simulink library "tqd"  (R2021b)
settings: Solver=VariableStepAuto  StartTime=0.0  StopTime=10.0  RelTol=1e-3
undefined symbols (not defined in the file): ATQD_AfterTqMinGain_X_Deg, ATQD_APSCreepBaseTqD_X_kph, ATQD_APSCreepBaseTqD_Y_Deg, ATQD_APSCreepBaseTqR_X_kph, ATQD_APSCreepBaseTqR_Y_Deg, ATQD_APSCreepIterm_X_kph, ATQD_APSCreepIterm_Y_kph, ATQD_APSCreepPterm_X_kph, ATQD_APSCreepPterm_Y_kph, ATQD_APSDecReq_X_kph, ATQD_APSDecReq_Y_mps2, ATQD_APSDecReqCMD_X_kph, ATQD_APSDecReqTs_X_pct, ATQD_APSDecTimeGain_X_Deg, ATQD_APSDecTimeGain_Y_s, ATQD_APSReqLowSpd_X_Deg, ATQD_AutoHoldReleaseBPS_X_Deg, ATQD_AWDLoadTrqnsGain_X_kg, ATQD_AWDLoadTrqnsGain_Y_pct, ATQD_BOSEnBPSPosn_X_kph, ATQD_BOSMap_X_rpm, ATQD_BOSMap_Y_pct, ATQD_CreepBaseTqD_X_kph, ATQD_CreepBaseTqD_Y_Deg, ATQD_CreepBaseTqR_X_kph, ATQD_CreepBaseTqR_Y_Deg, ATQD_CreepBPSDisPosn_X_Deg, ATQD_CreepBPSDisPosnR_X_Deg, ATQD_CreepBPSEnPosn_X_Deg, ATQD_CreepBPSEnPosnR_X_Deg, ATQD_CreepDeltaTq_X_kph, ATQD_CreepIterm_X_kph, ATQD_CreepIterm_Y_kph, ATQD_CreepItermMaxLimit_X_pct, ATQD_CreepPreloadTime_X_kph, ATQD_CreepPreloadTq_X_kph, ATQD_CreepPreloadTq_Y_s, ATQD_CreepProtTq_X_Deg, ATQD_CreepPterm_X_kph, ATQD_CreepPterm_Y_kph, ATQD_CreepRrTqSpRat_X_rpm, ATQD_CreepRrTqSpRat_Y_Nm, ATQD_CreepTargetSpdD_X_pct, ATQD_CreepTargetSpdR_X_pct, ATQD_ECOTqMapD_X_rpm, ATQD_ECOTqMapD_Y_pct, ATQD_EMTqMapD_X_rpm, ATQD_EMTqMapD_Y_pct, ATQD_EOPDTqMapDCon_X_rpm, ATQD_EOPDTqMapDCon_Y_Deg, ATQD_EscapeModePedTq_X_pct, ATQD_EscapeModePedTq_Y_rpm, ATQD_EscapeModePedTqFr_X_pct, ATQD_EscapeModePedTqFr_Y_rpm, ATQD_EstInitVehWeight_X_c, ATQD_FAfterTqCMDGain_X_rpm, ATQD_FAfterTqCMDGain_Y_pct, ATQD_FrLossMAPLowV_X_rpm, ATQD_FrLossMAPLowV_Y_Nm, ATQD_FrMotActReduce_X_rpm ... (+772)
libraries: simulink x211, hcu_lib x179, tqr x3
(part 13 of 28)

== system tqd/TQD/TorqueDemand/Signal_convert/VehWeightEst/Condition ==
  VTQD_AfterAvailableTqDemRr_Nm : Inport
  VTQR_NoABSREDUWhlTqReq_Nm : Inport  Port=2
  VTQR_NoABSFEDUWhlTqReq_Nm : Inport  Port=3
  VTQD_AfterAvailableTqDemFr_Nm : Inport  Port=4
  VTQD_GearActualPosn_enum : Inport  Port=5
  VINP_VehSpeed_kph : Inport  Port=6
  VTQD_RollRegenDisableReq_flg : Inport  Port=7
  VINP_RegenMode_enum : Inport  Port=8
  VTQD_LowIdleAccPedal_flg : Inport  Port=9
  VTQD_BrkSwSta_flg : Inport  Port=10
  VINP_RrRBCActive_flg : Inport  Port=11
  VINP_FrRBCActive_flg : Inport  Port=12
  VINP_GRADE_Deg : Inport  Port=13
  task_time_s : Inport  Port=14
  VTQD_VehWeightEstEnd_flg : Inport  Port=15
  AND1 : Logic  Inputs=13  AllPortsSameDT=off  OutDataTypeStr=boolean
  Abs : Abs
  Abs1 : Abs
  Abs2 : Abs
  Add : Sum  Inputs=+-
  Add1 : Sum  Inputs=+-
  Constant1 : Constant  Value=KTQD_VehWeightEstSpdEnLow_kph
  Constant10 : Constant  Value=eps
  Constant11 : Constant  Value=KTQD_VehWeightEstSpdEnUp_kph
  Constant2 : Constant  Value=ENUM_REGENLEVEL_LV1
  Constant3 : Constant  Value=KTQD_RrTqDeviation_Nm
  Constant4 : Constant  Value=KTQD_FrTqDeviation_Nm
  Constant5 : Constant  Value=KTQD_VehWeightEstGradeEn_Deg
  Constant6 : Constant  Value=KTQD_VehWeighEstTime_s
  Constant7 : Constant  Value=KTQD_EstDelayEnTime_s
  Constant8 : Constant  Value=KTQD_EstWeighResetTime_s
  Constant9 : Constant  Value=ENUM_GEARACTUALPOSN_D
  Delay{,1..5} (6 alike) : Delay  DelayLength=1
  DelayEnable : hcu_lib/Basic_Blocks/DelayEnable
  Detect Increase : simulink/Logic and Bit Operations/Detect Increase  vinit=0.0  OutDataTypeStr=boolean
  Equal : RelationalOperator  Operator=<  OutDataTypeStr=boolean  RndMeth=Simplest
  Equal1 : RelationalOperator  Operator===  OutDataTypeStr=boolean  RndMeth=Simplest
  Equal2 : RelationalOperator  Operator=~=  OutDataTypeStr=boolean  RndMeth=Simplest
  Less Than1 : RelationalOperator  Operator=<  OutDataTypeStr=boolean  RndMeth=Simplest
  Less Than2 : RelationalOperator  Operator=>  OutDataTypeStr=boolean  RndMeth=Simplest
  Less Than3 : RelationalOperator  Operator=<=  OutDataTypeStr=boolean  RndMeth=Simplest
  Less Than4 : RelationalOperator  Operator=<=  OutDataTypeStr=boolean  RndMeth=Simplest
  Less Than5 : RelationalOperator  Operator=<=  OutDataTypeStr=boolean  RndMeth=Simplest
  NOT{,1..5} (6 alike) : Logic  Operator=NOT  AllPortsSameDT=off  OutDataTypeStr=boolean
  Relational Operator : RelationalOperator  OutDataTypeStr=boolean  RndMeth=Simplest
  Relational Operator1 : RelationalOperator  OutDataTypeStr=boolean  RndMeth=Simplest
  SR_Latch : hcu_lib/Basic_Blocks/SR_Latch
  Timer : hcu_lib/Basic_Blocks/Timer
  Timer1 : hcu_lib/Basic_Blocks/Timer
  VTQD_VehWeightEstEn_flg : Outport
  VTQD_VehWeightEstDis_flg : Outport  Port=2
  wires:
  Constant9/1 -> Equal1/2
  Less Than1/1 -> AND1/2  "VTQD_VehWeightEstEnCon2_flg"
  Abs/1 -> [VTQD_RrTqErr_Nm]  "VTQD_RrTqErr_Nm"
  Equal1/1 -> AND1/1  "VTQD_VehWeightEstEnCon1_flg"
  Constant11/1 -> Less Than1/2
  [VTQR_NoABSFEDUWhlTqReq_Nm] -> Delay1/1
  Constant4/1 -> Less Than4/2
  Add1/1 -> Abs1/1
  [VTQD_RollRegenDisableReq_flg] -> NOT/1
  [VTQD_RrTqErr_Nm] -> Less Than3/1
  Add/1 -> Abs/1
  [VTQD_BrkSwSta_flg] -> NOT3/1
  [VTQD_FrTqErr_Nm] -> Less Than4/1
  Abs1/1 -> [VTQD_FrTqErr_Nm]  "VTQD_FrTqErr_Nm"
  [VTQD_GearActualPosn_enum] -> Equal1/1
  [VINP_VehSpeed_kph] -> Less Than1/1
  [VINP_RegenMode_enum] -> Equal2/1
  [VTQD_AfterAvailableTqDemFr_Nm] -> Delay4/1
  Constant1/1 -> Less Than2/2
  [VTQD_AfterAvailableTqDemRr_Nm] -> Delay2/1
  Less Than4/1 -> AND1/8  "VTQD_VehWeightEstEnCon7_flg"
  [VINP_RrRBCActive_flg] -> NOT4/1
  [VTQR_NoABSREDUWhlTqReq_Nm] -> Delay3/1
  NOT/1 -> AND1/4  "VTQD_VehWeightEstEnCon4_flg"
  [VINP_FrRBCActive_flg] -> NOT5/1
  Constant5/1 -> Less Than5/2
  Equal2/1 -> AND1/5  "VTQD_VehWeightEstEnCon5_flg"
  [VTQD_LowIdleAccPedal_flg] -> AND1/6
  Constant2/1 -> Equal2/2
  Less Than3/1 -> AND1/7  "VTQD_VehWeightEstEnCon6_flg"
  Less Than2/1 -> AND1/3  "VTQD_VehWeightEstEnCon3_flg"
  [VINP_VehSpeed_kph] -> Less Than2/1
  Less Than5/1 -> AND1/12  "VTQD_VehWeightEstEnCon11_flg"
  [VINP_GRADE_Deg] -> Abs2/1
  Abs2/1 -> Less Than5/1
  Constant3/1 -> Less Than3/2
  VTQD_AfterAvailableTqDemRr_Nm/1 -> [VTQD_AfterAvailableTqDemRr_Nm]
  VTQR_NoABSREDUWhlTqReq_Nm/1 -> [VTQR_NoABSREDUWhlTqReq_Nm]
  VTQD_AfterAvailableTqDemFr_Nm/1 -> [VTQD_AfterAvailableTqDemFr_Nm]
  VTQR_NoABSFEDUWhlTqReq_Nm/1 -> [VTQR_NoABSFEDUWhlTqReq_Nm]
  VTQD_GearActualPosn_enum/1 -> [VTQD_GearActualPosn_enum]
  VINP_VehSpeed_kph/1 -> [VINP_VehSpeed_kph]
  VTQD_RollRegenDisableReq_flg/1 -> [VTQD_RollRegenDisableReq_flg]
  VINP_RegenMode_enum/1 -> [VINP_RegenMode_enum]
  VTQD_LowIdleAccPedal_flg/1 -> [VTQD_LowIdleAccPedal_flg]
  VTQD_BrkSwSta_flg/1 -> [VTQD_BrkSwSta_flg]
  VINP_RrRBCActive_flg/1 -> [VINP_RrRBCActive_flg]
  VINP_FrRBCActive_flg/1 -> [VINP_FrRBCActive_flg]
  VINP_GRADE_Deg/1 -> [VINP_GRADE_Deg]
  [VTQD_VehWeightEstEn_flg] -> VTQD_VehWeightEstEn_flg/1
  Relational Operator/1 -> [VTQD_VehWeightEstDis_flg]  "VTQD_VehWeightEstDis_flg"
  Timer/1 -> Relational Operator/1
  NOT1/1 -> Timer/2
  [VTQD_VehWeightEstEn_flg] -> NOT1/1, Timer/1
  Constant6/1 -> Relational Operator/2, Timer/4
  [VTQD_VehWeightEstDis_flg] -> VTQD_VehWeightEstDis_flg/1
  task_time_s/1 -> [task_time_s]
  AND1/1 -> DelayEnable/1
  DelayEnable/1 -> [VTQD_VehWeightEstEn_flg]  "VTQD_VehWeightEstEn_flg"
  [task_time_s] -> DelayEnable/3
  Constant7/1 -> DelayEnable/2
  [VTQD_VehWeightEstEnd_flg] -> Detect Increase/1
  Detect Increase/1 -> SR_Latch/1
  SR_Latch/1 -> NOT2/1, Timer1/1
  NOT2/1 -> Timer1/2
  Constant8/1 -> Relational Operator1/2, Timer1/4
  Timer1/1 -> [VTQD_EstVehWeightResetTime_s], Relational Operator1/1  "VTQD_EstVehWeightResetTime_s"
  Relational Operator1/1 -> [VTQD_EstVehWeitResetFinish_flg]  "VTQD_EstVehWeitResetFinish_flg"
  [VTQD_EstVehWeitResetFinish_flg] -> Delay/1
  Delay/1 -> SR_Latch/2
  [VTQD_EstVehWeightResetTime_s] -> Delay5/1
  Constant10/1 -> Equal/2
  Equal/1 -> AND1/13  "VTQD_VehWeightEstEnCon12_flg"
  VTQD_VehWeightEstEnd_flg/1 -> [VTQD_VehWeightEstEnd_flg]
  Delay1/1 -> Add1/1
  Delay2/1 -> Add/1
  Delay3/1 -> Add/2
  Delay4/1 -> Add1/2
  Delay5/1 -> Equal/1
  NOT3/1 -> AND1/9  "VTQD_VehWeightEstEnCon8_flg"
  NOT4/1 -> AND1/10  "VTQD_VehWeightEstEnCon9_flg"
  NOT5/1 -> AND1/11  "VTQD_VehWeightEstEnCon10_flg"
  [task_time_s] -> Timer/3
  [task_time_s] -> Timer1/3

== system tqd/TQD/TorqueDemand/Signal_convert/VehWeightEst/Desicion ==
  task_time_s : Inport
  VTQD_VehWeightEstDis_flg : Inport  Port=2
  VTQD_EstVehWeight_kg : Inport  Port=3
  VINP_DriverSeatBeltCmd_flg : Inport  Port=4
  VINP_PsngrSeatBeltCmd_flg : Inport  Port=5
  VINP_RDriverSeatBeltCmd_flg : Inport  Port=6
  VINP_RCenterSeatBeltCmd_flg : Inport  Port=7
  VINP_RPsngrSeatBeltCmd_flg : Inport  Port=8
  VTQD_EstLongAccCheckPass_flg : Inport  Port=9
  VTQD_EstFrRealTqCheckPass_flg : Inport  Port=10
  VTQD_EstRrRealTqCheckPass_flg : Inport  Port=11
  AND : Logic  Inputs=5  AllPortsSameDT=off  OutDataTypeStr=boolean
  Add : Sum  Inputs=+++++
  Constant1 : Constant  Value=eps
  Constant{2,4,6,8,10} (5 alike) : Constant  Value=ZERO_INT
  Constant{3,5,7,9,11} (5 alike) : Constant  Value=ONE_INT
  Constant12 : Constant  Value=KTQD_EstEndDelayTime_s
  Data Type Conversion : DataTypeConversion  OutDataTypeStr=single
  Delay : Delay  DelayLength=1
  Delay1 : Delay  DelayLength=1
  DelayEnable : hcu_lib/Basic_Blocks/DelayEnable
  Equal : RelationalOperator  OutDataTypeStr=boolean  RndMeth=Simplest
  MTQD_EstInitVehWeight_Y_kg : Lookup_n-D  NumberOfTableDimensions=1  BreakpointsForDimension1=ATQD_EstInitVehWeight_X_c  Table=MTQD_EstInitVehWeight_Y_kg  ExtrapMethod=Clip  InternalRulePriority=Speed  RndMeth=Simplest  InputSameDT=on
  NOT : Logic  Operator=NOT  AllPortsSameDT=off  OutDataTypeStr=boolean
  Switch{,1..6} (7 alike) : Switch  Criteria=u2 > Threshold
  VTQD_VehWeightEstEnd_flg : Outport
  VTQD_EstVehWeightResult_kg : Outport  Port=2
  wires:
  Constant7/1 -> Switch4/1
  Constant1/1 -> Equal/2
  Switch2/1 -> Add/1
  [VINP_DriverSeatBeltCmd_flg] -> Switch2/2
  [VINP_RCenterSeatBeltCmd_flg] -> Switch4/2
  Switch5/1 -> Add/4
  Equal/1 -> Switch1/2
  Constant10/1 -> Switch6/3
  [VTQD_VehWeightEstDis_flg] -> AND/1
  Switch6/1 -> Add/5
  Delay/1 -> NOT/1
  Switch3/1 -> Add/2
  Constant6/1 -> Switch4/3
  Constant3/1 -> Switch2/1
  [VTQD_EstActVehWeight_kg] -> Switch1/1
  Constant2/1 -> Switch2/3
  [VTQD_VehWeightEstEnter_flg] -> Switch/2
  Constant11/1 -> Switch6/1
  Switch1/1 -> [VTQD_EstVehWeightResult_kg]  "VTQD_EstVehWeightResult_kg"
  Constant4/1 -> Switch3/3
  Constant5/1 -> Switch3/1
  [VINP_RDriverSeatBeltCmd_flg] -> Switch5/2
  Switch/1 -> Delay1/1, [VTQD_EstActVehWeight_kg]  "VTQD_EstActVehWeight_kg"
  AND/1 -> [VTQD_VehWeightEstEnter_flg]  "VTQD_VehWeightEstEnter_flg"
  [VINP_RPsngrSeatBeltCmd_flg] -> Switch6/2
  [VTQD_EstActVehWeight_kg] -> Equal/1
  [VINP_PsngrSeatBeltCmd_flg] -> Switch3/2
  Delay1/1 -> Switch/3
  [VTQD_EstInitVehWeight_kg] -> Switch1/3
  Constant9/1 -> Switch5/1
  Constant8/1 -> Switch5/3
  [VTQD_EstVehWeight_kg] -> Switch/1
  [VTQD_VehWeightEstEnd_flg] -> Delay/1
  NOT/1 -> AND/2
  Switch4/1 -> Add/3
  [VTQD_VehWeightEstDis_flg] -> DelayEnable/1
  Constant12/1 -> DelayEnable/2
  [task_time_s] -> DelayEnable/3
  DelayEnable/1 -> [VTQD_VehWeightEstEnd_flg]  "VTQD_VehWeightEstEnd_flg"
  task_time_s/1 -> [task_time_s]
  [VTQD_VehWeightEstEnd_flg] -> VTQD_VehWeightEstEnd_flg/1
  VTQD_VehWeightEstDis_flg/1 -> [VTQD_VehWeightEstDis_flg]
  VTQD_EstVehWeight_kg/1 -> [VTQD_EstVehWeight_kg]
  [VTQD_EstVehWeightResult_kg] -> VTQD_EstVehWeightResult_kg/1
  VINP_DriverSeatBeltCmd_flg/1 -> [VINP_DriverSeatBeltCmd_flg]
  VINP_PsngrSeatBeltCmd_flg/1 -> [VINP_PsngrSeatBeltCmd_flg]
  VINP_RDriverSeatBeltCmd_flg/1 -> [VINP_RDriverSeatBeltCmd_flg]
  VINP_RCenterSeatBeltCmd_flg/1 -> [VINP_RCenterSeatBeltCmd_flg]
  VINP_RPsngrSeatBeltCmd_flg/1 -> [VINP_RPsngrSeatBeltCmd_flg]
  VTQD_EstRrRealTqCheckPass_flg/1 -> [VTQD_EstRrRealTqCheckPass_flg]
  VTQD_EstFrRealTqCheckPass_flg/1 -> [VTQD_EstFrRealTqCheckPass_flg]
  VTQD_EstLongAccCheckPass_flg/1 -> [VTQD_EstLongAccCheckPass_flg]
  [VTQD_EstLongAccCheckPass_flg] -> AND/3
  [VTQD_EstFrRealTqCheckPass_flg] -> AND/4
  [VTQD_EstRrRealTqCheckPass_flg] -> AND/5
  MTQD_EstInitVehWeight_Y_kg/1 -> [VTQD_EstInitVehWeight_kg]  "VTQD_EstInitVehWeight_kg"
  Data Type Conversion/1 -> MTQD_EstInitVehWeight_Y_kg/1
  Add/1 -> Data Type Conversion/1  "VTQD_EstInitVehWightX_c"

== system tqd/TQD/TorqueDemand/TorqueModule/AvaliableTqLimit/If Action Subsystem1 ==
  VTQD_WhlTqCapGenF_Nm : Inport
  VTQD_WhlTqCapGenR_Nm : Inport  Port=2
  VTQD_DriverWhlTqDemFr_Nm : Inport  Port=3
  VTQD_DriverWhlTqDemRr_Nm : Inport  Port=4
  VVMC_ADASActive_flg : Inport  Port=5
  Action Port : ActionPort
  Constant{,1..3} (4 alike) : Constant  Value=ZERO_FLOAT
  Data Type Conversion1 : DataTypeConversion  OutDataTypeStr=single
  Data Type Conversion5 : DataTypeConversion  OutDataTypeStr=single
  Display : Display
  Display1 : Display
  Subtract : Sum  Inputs=+-
  Subtract1 : Sum  Inputs=+-
  Switch : Switch  Criteria=u2 > Threshold
  Switch1 : Switch  Criteria=u2 > Threshold
  Switch2 : Switch  Criteria=u2 ~= 0
  Switch3 : Switch  Criteria=u2 ~= 0
  VTQD_AvailTqWithARgnFr_Nm : Outport
  VTQD_AvailTqWithARgnRr_Nm : Outport  Port=2
  wires:
  Constant1/1 -> Switch1/1
  Constant/1 -> Switch/1
  Subtract1/1 -> Switch1/2, Switch1/3
  Subtract/1 -> Switch/2, Switch/3
  Switch1/1 -> Data Type Conversion5/1, VTQD_AvailTqWithARgnRr_Nm/1
  Switch/1 -> Data Type Conversion1/1, VTQD_AvailTqWithARgnFr_Nm/1
  VTQD_WhlTqCapGenR_Nm/1 -> Subtract1/1
  VTQD_WhlTqCapGenF_Nm/1 -> Subtract/1
  VTQD_DriverWhlTqDemFr_Nm/1 -> Switch2/3
  Switch2/1 -> Subtract/2
  Constant2/1 -> Switch2/1
  VVMC_ADASActive_flg/1 -> Switch3/2, Switch2/2
  Constant3/1 -> Switch3/1
  VTQD_DriverWhlTqDemRr_Nm/1 -> Switch3/3
  Switch3/1 -> Subtract1/2
  Data Type Conversion1/1 -> Display/1  "VTQD_AvailTqWithARgnFr_Nm"
  Data Type Conversion5/1 -> Display1/1  "VTQD_AvailTqWithARgnRr_Nm"

== system tqd/TQD/TorqueDemand/TorqueModule/AvaliableTqLimit/If Action Subsystem2 ==
  VTQD_WhlTqCapGenF_Nm : Inport
  VTQD_WhlTqCapGenR_Nm : Inport  Port=2
  Action Port : ActionPort
  Data Type Conversion4 : DataTypeConversion  OutDataTypeStr=single
  Data Type Conversion5 : DataTypeConversion  OutDataTypeStr=single
  Display : Display
  Display1 : Display
  VTQD_AvailTqNoARgnFr_Nm : Outport
  VTQD_AvailTqNoARgnRr_Nm : Outport  Port=2
  wires:
  VTQD_WhlTqCapGenF_Nm/1 -> Data Type Conversion4/1, VTQD_AvailTqNoARgnFr_Nm/1
  VTQD_WhlTqCapGenR_Nm/1 -> Data Type Conversion5/1, VTQD_AvailTqNoARgnRr_Nm/1
  Data Type Conversion4/1 -> Display/1  "VTQD_AvailTqNoARgnFr_Nm"
  Data Type Conversion5/1 -> Display1/1  "VTQD_AvailTqNoARgnRr_Nm"

== system tqd/TQD/TorqueDemand/TorqueModule/AvaliableTqLimit/TorqueCapacityCalcalation ==
  VTQD_FrShaftSpd_rpm : Inport
  VTQD_RrShaftSpd_rpm : Inport  Port=2
  VINP_HVBPwrAvailDchrg_kw : Inport  Port=3
  VINP_HVBPwrAvailChrg_kw : Inport  Port=4
  KTQD_FrBatapCont_factor : Inport  Port=5
  KTQD_RrBatapCont_factor : Inport  Port=6
  VTQD_FrEDUSpRat_cmd : Inport  Port=7
  VTQD_RrEDUSpRat_rat : Inport  Port=8
  VINP_FrMotorAvailTq_Nm : Inport  Port=9
  VINP_RrMotorAvailTq_Nm : Inport  Port=10
  VINP_FrRegenAvailTq_Nm : Inport  Port=11
  VINP_RrRegenAvailTq_Nm : Inport  Port=12
  VTQD_GearActualPosn_enum : Inport  Port=13
  VINP_VehicleType_enum : Inport  Port=14
  VTQD_CoordWhlTqDemFr_Nm : Inport  Port=15
  VTQD_CoordWhlTqDemRr_Nm : Inport  Port=16
  VINP_FrMCUDCBusVolt_V : Inport  Port=17
  VINP_RrMCUDCBusVolt_V : Inport  Port=18
  VPMM_DrivetrainSelect_enum : Inport  Port=19
  VINP_FrMCUTemp_C : Inport  Port=20
  VINP_FrTMTemp_C : Inport  Port=21
  VINP_RrMCUTemp_C : Inport  Port=22
  VINP_RrTMTemp_C : Inport  Port=23
  VTQD_IVIRockModeEn_flg : Inport  Port=24
  VTQD_ActAPSPosn_pct : Inport  Port=25
  task_time_s : Inport  Port=26
  CapacityDistribution : Subsystem
  Constant1 : Constant  Value=KTQD_RockInitMotTqInc_Nm
  Constant10 : Constant  Value=KTQD_RrUppTheldTrq_Nm
  Constant11 : Constant  Value=KTQD_RrUppTheldTrq_Nm
  Constant12 : Constant  Value=KTQD_RockInitTqMotDec_Nm
  Constant13 : Constant  Value=KTQD_RockAvalMotTqReset_pct
  Constant14 : Constant  Value=KTQD_RockAvalMotTqReset_pct
  Constant2 : Constant  Value=KTQD_FrRockAvalMotTqInc_Nm
  Constant3 : Constant  Value=KTQD_FrRockAvalMotBaseTq_Nm
  Constant4 : Constant  Value=KTQD_FrUppTheldTrq_Nm
  Constant5 : Constant  Value=KTQD_FrUppTheldTrq_Nm
  Constant6 : Constant  Value=KTQD_RockInitTqMotDec_Nm
  Constant7 : Constant  Value=KTQD_RockInitMotTqInc_Nm
  Constant8 : Constant  Value=KTQD_RrRockAvalMotTqInc_Nm
  Constant9 : Constant  Value=KTQD_RrRockAvalMotBaseTq_Nm
  Generation : Subsystem
  KTQD_FrMotorTempHigh_C KTQD_FrMotorTempLow_C : Relay  OnSwitchValue=KTQD_FrMotorTempHigh_C  OffSwitchValue=KTQD_FrMotorTempLow_C  OutDataTypeStr=boolean
  KTQD_RrMotorTempHigh_C KTQD_RrMotorTempLow_C : Relay  OnSwitchValue=KTQD_RrMotorTempHigh_C  OffSwitchValue=KTQD_RrMotorTempLow_C  OutDataTypeStr=boolean
  "MOTOR Loss MAP " : Subsystem
  MTQD_FrGenActReduce_Z_Nm : Lookup_n-D  BreakpointsForDimension1=ATQD_FrMotActReduce_Y_C  BreakpointsForDimension2=ATQD_FrMotActReduce_X_rpm  Table=MTQD_FrGenActReduce_Z_Nm  InternalRulePriority=Speed  RndMeth=Simplest  InputSameDT=on
      settings: InputPortMap=u0,u1
  MTQD_FrMotActReduce_Z_Nm : Lookup_n-D  BreakpointsForDimension1=ATQD_FrMotActReduce_Y_C  BreakpointsForDimension2=ATQD_FrMotActReduce_X_rpm  Table=MTQD_FrMotActReduce_Z_Nm  InternalRulePriority=Speed  RndMeth=Simplest  InputSameDT=on
      settings: InputPortMap=u0,u1
  MTQD_RrGenActReduce_Z_Nm : Lookup_n-D  BreakpointsForDimension1=ATQD_FrMotActReduce_Y_C  BreakpointsForDimension2=ATQD_FrMotActReduce_X_rpm  Table=MTQD_RrGenActReduce_Z_Nm  InternalRulePriority=Speed  RndMeth=Simplest  InputSameDT=on
      settings: InputPortMap=u0,u1
  MTQD_RrMotActReduce_Z_Nm : Lookup_n-D  BreakpointsForDimension1=ATQD_FrMotActReduce_Y_C  BreakpointsForDimension2=ATQD_FrMotActReduce_X_rpm  Table=MTQD_RrMotActReduce_Z_Nm  InternalRulePriority=Speed  RndMeth=Simplest  InputSameDT=on
      settings: InputPortMap=u0,u1
  Max{,1..7} (8 alike) : MinMax  Function=max  Inputs=2
  Motoring : Subsystem
  OR : Logic  Operator=OR  AllPortsSameDT=off  OutDataTypeStr=boolean
  OR1 : Logic  Operator=OR  AllPortsSameDT=off  OutDataTypeStr=boolean
  RateLimit : hcu_lib/Basic_Blocks/RateLimit
  RateLimit1 : hcu_lib/Basic_Blocks/RateLimit
  Relational Operator : RelationalOperator  Operator=<=  OutDataTypeStr=boolean  RndMeth=Simplest
  Relational Operator1 : RelationalOperator  Operator=<=  OutDataTypeStr=boolean  RndMeth=Simplest
  Switch{,1..3} (4 alike) : Switch  Criteria=u2 ~= 0
      settings: AttributesFormatString=%<Criteria>
  TMAvailablePwr_Calculation : Subsystem
  VTQD_WhlTqCapMotFr_Nm : Outport
  VTQD_WhlTqCapMotRr_Nm : Outport  Port=2
  VTQD_WhlTqCapGenFr_Nm : Outport  Port=3
  VTQD_WhlTqCapGenRr_Nm : Outport  Port=4
  VTQD_MotorLossTotal_kw : Outport  Port=5
  wires:
  [VTQD_TMPwrAvailDchrg_kW] -> CapacityDistribution/3(VTQD_TMPwrAvailDchrg_kW)
  TMAvailablePwr_Calculation/1(VTQD_TMPwrAvailDchrg_kW) -> [VTQD_TMPwrAvailDchrg_kW]
  [VINP_HVBPwrAvailDchrg_kw] -> TMAvailablePwr_Calculation/1(VINP_HVBPwrAvailDchrg_kw)
  Motoring/2(VTQD_WhlTqCapMotRr_Nm) -> VTQD_WhlTqCapMotRr_Nm/1
  [VTQD_RrEDUSpRat_rat] -> CapacityDistribution/2(VTQD_RrEDUSpRat_rat)
  [VTQD_FrEDUSpRat_rat] -> CapacityDistribution/1(VTQD_FrEDUSpRat_cmd)
  CapacityDistribution/4(VTQD_RrHVBPwrAvailChrg_kw) -> [VTQD_RrHVBPwrAvailChrg_kw]
  CapacityDistribution/3(VTQD_FrHVBPwrAvailChrg_kw) -> [VTQD_FrHVBPwrAvailChrg_kw]
  CapacityDistribution/2(VTQD_RrHVBPwrAvailDchrg_kw) -> [VTQD_RrHVBPwrAvailDchrg_kw]
  CapacityDistribution/1(VTQD_FrHVBPwrAvailDchrg_kw) -> [VTQD_FrHVBPwrAvailDchrg_kw]
  [VINP_HVBPwrAvailChrg_kw] -> CapacityDistribution/4(VINP_HVBPwrAvailChrg_kw)
  [VTQD_RrHVBPwrAvailChrg_kw] -> Generation/4(VTQD_RrHVBPwrAvailChrg_kw)
  [KTQD_RrBatapCont_factor] -> Generation/6(KTQD_RrBatapCont_factor)
  [VTQD_FrShaftSpd_rpm] -> Generation/1(VTQD_FrShaftSpd_rpm)
  [VTQD_FrHVBPwrAvailChrg_kw] -> Generation/3(VTQD_FrHVBPwrAvailChrg_kw)
  [VTQD_RrShaftSpd_rpm] -> Generation/2(VTQD_RrShaftSpd_rpm)
  [KTQD_FrBatapCont_factor] -> Generation/5(KTQD_FrBatapCont_factor)
  Generation/1(VTQD_WhlTqCapGenFr_Nm) -> VTQD_WhlTqCapGenFr_Nm/1
  Generation/2(VTQD_WhlTqCapGenRr_Nm) -> VTQD_WhlTqCapGenRr_Nm/1
  [VTQD_RrHVBPwrAvailDchrg_kw] -> Motoring/4(VTQD_RrHVBPwrAvailDchrg_kw)
  [VTQD_FrHVBPwrAvailDchrg_kw] -> Motoring/3(VTQD_FrHVBPwrAvailDchrg_kw)
  [KTQD_RrBatapCont_factor] -> Motoring/6(KTQD_RrBatapCont_factor)
  VTQD_RrEDUSpRat_rat/1 -> [VTQD_RrEDUSpRat_rat]
  VTQD_FrEDUSpRat_cmd/1 -> [VTQD_FrEDUSpRat_rat]
  KTQD_RrBatapCont_factor/1 -> [KTQD_RrBatapCont_factor]
  [VTQD_RrShaftSpd_rpm] -> Motoring/2(VTQD_RrShaftSpd_rpm)
  VTQD_RrShaftSpd_rpm/1 -> [VTQD_RrShaftSpd_rpm]
  VTQD_FrShaftSpd_rpm/1 -> [VTQD_FrShaftSpd_rpm]
  VINP_HVBPwrAvailChrg_kw/1 -> [VINP_HVBPwrAvailChrg_kw]
  VINP_HVBPwrAvailDchrg_kw/1 -> [VINP_HVBPwrAvailDchrg_kw]
  KTQD_FrBatapCont_factor/1 -> [KTQD_FrBatapCont_factor]
  [VTQD_FrShaftSpd_rpm] -> Motoring/1(VTQD_FrShaftSpd_rpm)
  Motoring/1(VTQD_WhlTqCapMotFr_Nm) -> VTQD_WhlTqCapMotFr_Nm/1
  [KTQD_FrBatapCont_factor] -> Motoring/5(KTQD_FrBatapCont_factor)
  [VINP_RrMotorAvailTq_Nm] -> Motoring/8(VINP_RrMotorAvailTq_Nm)
  [VINP_FrMotorAvailTq_Nm] -> Motoring/7(VINP_FrMotorAvailTq_Nm)
  [VINP_FrRegenAvailTq_Nm] -> Generation/7(VINP_FrRegenAvailTq_Nm)
  [VINP_RrRegenAvailTq_Nm] -> Generation/8(VINP_RrRegenAvailTq_Nm)
  VINP_RrRegenAvailTq_Nm/1 -> [VINP_RrRegenAvailTq_Nm]
  VINP_FrRegenAvailTq_Nm/1 -> [VINP_FrRegenAvailTq_Nm]
  VINP_FrMotorAvailTq_Nm/1 -> [VINP_FrMotorAvailTq_Nm]
  VINP_RrMotorAvailTq_Nm/1 -> [VINP_RrMotorAvailTq_Nm]
  [VTQD_GearActualPosn_enum] -> Motoring/9(VTQD_GearActualPosn_enum)
  VTQD_GearActualPosn_enum/1 -> [VTQD_GearActualPosn_enum]
  [VTQD_GearActualPosn_enum] -> Generation/9(VTQD_GearActualPosn_enum)
  VINP_VehicleType_enum/1 -> [VINP_VehicleType_enum]
  [VINP_VehicleType_enum] -> Motoring/10(VINP_VehicleType_enum)
  [VINP_VehicleType_enum] -> Generation/10(VINP_VehicleType_enum)
  [VTQD_FrShaftSpd_rpm] -> "MOTOR Loss MAP "/1(VTQD_FrShaftSpd_rpm)
  [VTQD_RrShaftSpd_rpm] -> "MOTOR Loss MAP "/2(VTQD_RrShaftSpd_rpm)
  [VTQD_CoordWhlTqDemFr_Nm] -> "MOTOR Loss MAP "/3(VTQD_CoordWhlTqDemFr_Nm)
  [VTQD_CoordWhlTqDemRr_Nm] -> "MOTOR Loss MAP "/4(VTQD_CoordWhlTqDemRr_Nm)
  [VINP_FrMCUDCBusVolt_V] -> "MOTOR Loss MAP "/5(VINP_FrMCUDCBusVolt_V)
  [VINP_RrMCUDCBusVolt_V] -> "MOTOR Loss MAP "/6(VINP_RrMCUDCBusVolt_V)
  [VPMM_DrivetrainSelect_enum] -> "MOTOR Loss MAP "/7(VPMM_DrivetrainSelect_enum)
  VTQD_CoordWhlTqDemRr_Nm/1 -> [VTQD_CoordWhlTqDemRr_Nm]
  VTQD_CoordWhlTqDemFr_Nm/1 -> [VTQD_CoordWhlTqDemFr_Nm]
  VINP_FrMCUDCBusVolt_V/1 -> [VINP_FrMCUDCBusVolt_V]
  VINP_RrMCUDCBusVolt_V/1 -> [VINP_RrMCUDCBusVolt_V]
  VPMM_DrivetrainSelect_enum/1 -> [VPMM_DrivetrainSelect_enum]
  "MOTOR Loss MAP "/1(VTQD_MotorLossTotal_kw) -> VTQD_MotorLossTotal_kw/1, [VTQD_MotorLossTotal_kw]
  [VTQD_MotorLossTotal_kw] -> CapacityDistribution/5(VTQD_MotorLossTotal_kw)
  VINP_FrMCUTemp_C/1 -> [VINP_FrMCUTemp_C]
  VINP_FrTMTemp_C/1 -> [VINP_FrTMTemp_C]
  VINP_RrMCUTemp_C/1 -> [VINP_RrMCUTemp_C]
  VINP_RrTMTemp_C/1 -> [VINP_RrTMTemp_C]
  [VINP_FrMCUTemp_C] -> Max/1
  [VINP_FrTMTemp_C] -> Max/2
  Max/1 -> KTQD_FrMotorTempHigh_C KTQD_FrMotorTempLow_C/1
  KTQD_FrMotorTempHigh_C KTQD_FrMotorTempLow_C/1 -> [VTQD_FrMotorTempHigh_flg]  "VTQD_FrMotorTempHigh_flg"
  KTQD_RrMotorTempHigh_C KTQD_RrMotorTempLow_C/1 -> [VTQD_RrMotorTempHigh_flg]  "VTQD_RrMotorTempHigh_flg"
  Max1/1 -> KTQD_RrMotorTempHigh_C KTQD_RrMotorTempLow_C/1
  [VINP_RrTMTemp_C] -> Max1/2
  [VINP_RrMCUTemp_C] -> Max1/1
  MTQD_FrMotActReduce_Z_Nm/1 -> [VTQD_FrMotActReduce_Nm]  "VTQD_FrMotActReduce_Nm"
  MTQD_FrGenActReduce_Z_Nm/1 -> [VTQD_FrGenActReduce_Nm]  "VTQD_FrGenActReduce_Nm"
  [VTQD_FrShaftSpd_rpm] -> MTQD_FrGenActReduce_Z_Nm/2
  [VTQD_RrShaftSpd_rpm] -> MTQD_RrGenActReduce_Z_Nm/2
  MTQD_RrGenActReduce_Z_Nm/1 -> [VTQD_RrGenActReduce_Nm]  "VTQD_RrGenActReduce_Nm"
  MTQD_RrMotActReduce_Z_Nm/1 -> [VTQD_RrMotActReduce_Nm]  "VTQD_RrMotActReduce_Nm"
  [VTQD_RrShaftSpd_rpm] -> MTQD_RrMotActReduce_Z_Nm/2
  [VTQD_FrMotorTempHigh_flg] -> Motoring/11(VTQD_FrMotorTempHigh_flg)
  [VTQD_RrMotorTempHigh_flg] -> Motoring/12(VTQD_RrMotorTempHigh_flg)
  [VTQD_FrMotActReduce_Nm] -> Motoring/13(VTQD_FrMotActReduce_gain)
  [VTQD_RrMotActReduce_Nm] -> Motoring/14(VTQD_RrMotActReduce_Nm)
  [VTQD_RrGenActReduce_Nm] -> Generation/14(VTQD_RrGenActReduce_Nm)
  [VTQD_FrGenActReduce_Nm] -> Generation/13(VTQD_FrGenActReduce_Nm)
  [VTQD_FrMotorTempHigh_flg] -> Generation/11(VTQD_FrMotorTempHigh_flg)
  [VTQD_RrMotorTempHigh_flg] -> Generation/12(VTQD_RrMotorTempHigh_flg)
  [VINP_FrMCUTemp_C] -> Max2/1
  [VINP_FrTMTemp_C] -> Max2/2
  Max2/1 -> MTQD_FrMotActReduce_Z_Nm/1
  [VTQD_FrShaftSpd_rpm] -> MTQD_FrMotActReduce_Z_Nm/2
  [VINP_FrTMTemp_C] -> Max3/2
  [VINP_FrMCUTemp_C] -> Max3/1
  Max3/1 -> MTQD_FrGenActReduce_Z_Nm/1
  [VINP_RrMCUTemp_C] -> Max4/1
  [VINP_RrTMTemp_C] -> Max4/2
  Max4/1 -> MTQD_RrMotActReduce_Z_Nm/1
  [VINP_RrTMTemp_C] -> Max5/2
  [VINP_RrMCUTemp_C] -> Max5/1
  Max5/1 -> MTQD_RrGenActReduce_Z_Nm/1
  VTQD_IVIRockModeEn_flg/1 -> [VTQD_IVIRockModeEn_flg]
  [VTQD_CoordWhlTqDemFr_Nm] -> Max6/2
  Constant3/1 -> Max6/1
  Max6/1 -> Switch/1
  [VTQD_IVIRockModeEn_flg] -> Switch/2
  OR/1 -> Switch1/2
  [VTQD_IVIRockModeEn_flg] -> OR/1
  VTQD_ActAPSPosn_pct/1 -> [VTQD_ActAPSPosn_pct]
  Constant1/1 -> Switch1/1
  Constant2/1 -> Switch1/3
  Switch/1 -> [VTQD_FrRockDisAvalMotInpTq_Nm]  "VTQD_FrRockDisAvalMotInpTq_Nm"
  Switch1/1 -> [VTQD_FrRockAvalMotTqInc_Nm]  "VTQD_FrRockAvalMotTqInc_Nm"
  [VTQD_FrRockDisAvalMotInpTq_Nm] -> RateLimit/1
  Constant4/1 -> Switch/3
  Constant5/1 -> RateLimit/2
  task_time_s/1 -> [task_time_s]
  [task_time_s] -> RateLimit/3
  [VTQD_FrRockAvalMotTqInc_Nm] -> RateLimit/4
  Constant6/1 -> RateLimit/5
  RateLimit/1 -> [VTQD_FrRockDisAvalMotTq_Nm]  "VTQD_FrRockDisAvalMotTq_Nm"
  RateLimit1/1 -> [VTQD_RrRockDisAvalMotTq_Nm]  "VTQD_RrRockDisAvalMotTq_Nm"
  Constant12/1 -> RateLimit1/5
  [VTQD_RrRockAvalMotTqInc_Nm] -> RateLimit1/4
  [task_time_s] -> RateLimit1/3
  Constant11/1 -> RateLimit1/2
  Constant10/1 -> Switch2/3
  [VTQD_RrRockDisAvalMotInpTq_Nm] -> RateLimit1/1
  Switch3/1 -> [VTQD_RrRockAvalMotTqInc_Nm]  "VTQD_RrRockAvalMotTqInc_Nm"
  Switch2/1 -> [VTQD_RrRockDisAvalMotInpTq_Nm]  "VTQD_RrRockDisAvalMotInpTq_Nm"
  Constant8/1 -> Switch3/3
  Constant7/1 -> Switch3/1
  [VTQD_IVIRockModeEn_flg] -> Switch2/2
  Max7/1 -> Switch2/1
  Constant9/1 -> Max7/1
  [VTQD_CoordWhlTqDemRr_Nm] -> Max7/2
  Relational Operator/1 -> OR/2
  [VTQD_ActAPSPosn_pct] -> Relational Operator/1
  Constant13/1 -> Relational Operator/2
  [VTQD_ActAPSPosn_pct] -> Relational Operator1/1
  OR1/1 -> Switch3/2
  [VTQD_IVIRockModeEn_flg] -> OR1/1
  Constant14/1 -> Relational Operator1/2
  Relational Operator1/1 -> OR1/2
  [VTQD_FrRockDisAvalMotTq_Nm] -> Motoring/15(VTQD_FrRockDisAvalMotTq_Nm)
  [VTQD_RrRockDisAvalMotTq_Nm] -> Motoring/16(VTQD_RrRockDisAvalMotTq_Nm)

== system tqd/TQD/TorqueDemand/TorqueModule/DriverWhlTqDem/BOS ==
  VTQD_ActBPSPosn_pct : Inport
  VTQD_TqTargetShaftSpd_rpm : Inport  Port=2
  VTQD_VehActSpd_kph : Inport  Port=3
  VTQD_PedalMapWhlTq_Nm : Inport  Port=4
  VTQD_CreepBaseTqR_Nm : Inport  Port=5
  VTQD_CreepBaseTqD_Nm : Inport  Port=6
  VTQD_GearActualPosn_enum : Inport  Port=7
  VVMC_APSActive_flg : Inport  Port=8
  VTQD_LowIdleAccPedal_flg : Inport  Port=9
  VTQD_HighBPSPosn_flg : Inport  Port=10
  VTQD_BrkSwSta_flg : Inport  Port=11
  VTQD_LimpHomeAct_flg : Inport  Port=12
  AND : Logic  Inputs=4  AllPortsSameDT=off  OutDataTypeStr=boolean
  AND1 : Logic  AllPortsSameDT=off  OutDataTypeStr=boolean
  AND2 : Logic  AllPortsSameDT=off  OutDataTypeStr=boolean
  Constant1 : Constant  Value=KTQD_BOSEnPedalTq_Nm
  Constant18 : Constant  Value=ZERO_FLOAT
  Constant20 : Constant  Value=ENUM_GEARACTUALPOSN_R
  Constant3 : Constant  Value=ONE_PERCENT
  Constant96 : Constant  Value=KTQD_FailsafeActiveSW_flg
  Detect Change : simulink/Logic and Bit Operations/Detect Change  vinit=0  OutDataTypeStr=boolean
  Equal10 : RelationalOperator  Operator===  OutDataTypeStr=boolean  RndMeth=Simplest
  Logical Operator13 : Logic  AllPortsSameDT=off  OutDataTypeStr=boolean
  MTQD_BOSEnBPSPosn_Y_pct : Lookup_n-D  NumberOfTableDimensions=1  BreakpointsForDimension1=ATQD_BOSEnBPSPosn_X_kph  Table=MTQD_BOSEnBPSPosn_Y_pct  InternalRulePriority=Speed  RndMeth=Simplest  InputSameDT=on
  MTQD_BOSMap_Z_pct : Lookup_n-D  BreakpointsForDimension1=ATQD_BOSMap_Y_pct  BreakpointsForDimension2=ATQD_BOSMap_X_rpm  Table=MTQD_BOSMap_Z_pct  ExtrapMethod=Clip  InternalRulePriority=Speed  RndMeth=Simplest  InputSameDT=on
      settings: InputPortMap=u0,u1
  Max : MinMax  Function=max  Inputs=2
  NOT{,1..3} (4 alike) : Logic  Operator=NOT  AllPortsSameDT=off  OutDataTypeStr=boolean
  OR : Logic  Operator=OR  Inputs=3  AllPortsSameDT=off  OutDataTypeStr=boolean
  OR1 : Logic  Operator=OR  AllPortsSameDT=off  OutDataTypeStr=boolean
  OR2 : Logic  Operator=OR  AllPortsSameDT=off  OutDataTypeStr=boolean
  Product1 : Product  RndMeth=Zero
  Product2 : Product  RndMeth=Zero
  Product3 : Product  RndMeth=Zero
  Relational Operator : RelationalOperator  Operator=>  OutDataTypeStr=boolean  RndMeth=Simplest
  Relational Operator1 : RelationalOperator  Operator=>  OutDataTypeStr=boolean  RndMeth=Simplest
  Relational Operator2 : RelationalOperator  OutDataTypeStr=boolean  RndMeth=Simplest
  Relational Operator5 : RelationalOperator  Operator=>  OutDataTypeStr=boolean  RndMeth=Simplest
  SR_Latch : hcu_lib/Basic_Blocks/SR_Latch
  Switch7 : Switch  Criteria=u2 > Threshold
  Switch8 : Switch  Criteria=u2 > Threshold
  VTQD_BOSEnable_flg : Outport
  VTQD_BOSTq_Nm : Outport  Port=2
  wires:
  VTQD_TqTargetShaftSpd_rpm/1 -> [VTQD_TqTargetShaftSpd_rpm]
  [VTQD_ActBPSPosn_pct] -> MTQD_BOSMap_Z_pct/1
  [VTQD_TqTargetShaftSpd_rpm] -> MTQD_BOSMap_Z_pct/2
  Constant3/1 -> Product1/2
  Product1/1 -> [VTQD_BOSReduction_gain]  "VTQD_BOSReduction_gain"
  MTQD_BOSMap_Z_pct/1 -> Product1/1
  VTQD_ActBPSPosn_pct/1 -> [VTQD_ActBPSPosn_pct]
  Relational Operator/1 -> AND/1
  VTQD_VehActSpd_kph/1 -> [VTQD_VehActSpd_kph]
  [VTQD_VehActSpd_kph] -> MTQD_BOSEnBPSPosn_Y_pct/1
  MTQD_BOSEnBPSPosn_Y_pct/1 -> Relational Operator/2  "VTQD_BOSEnBPSPosn_pct"
  [VTQD_ActBPSPosn_pct] -> Relational Operator/1
  VTQD_PedalMapWhlTq_Nm/1 -> [VTQD_PedalMapWhlTq_Nm]
  Relational Operator1/1 -> AND/2
  [VTQD_PedalMapWhlTq_Nm] -> Relational Operator1/1
  Constant1/1 -> Relational Operator1/2
  [VTQD_PedalMapWhlTq_Nm] -> Product2/1
  [VTQD_BOSReduction_gain] -> Product2/2
  Product3/1 -> Max/2
  Switch8/1 -> VTQD_BOSTq_Nm/1, [VTQD_BOSTq_Nm]  "VTQD_BOSTq_Nm"
  [VTQD_CreepBaseTqR_Nm] -> Switch7/1
  Max/1 -> Switch8/1
  Product2/1 -> Switch8/3
  Equal10/1 -> Switch7/2
  [VTQD_PedalMapWhlTq_Nm] -> Product3/1
  [VTQD_BOSReduction_gain] -> Product3/2
  [VTQD_GearActualPosn_enum] -> Equal10/1
  Relational Operator5/1 -> Switch8/2
  Constant20/1 -> Equal10/2
  Switch7/1 -> Max/1
  Constant18/1 -> Relational Operator5/2
  [VTQD_CreepBaseTqD_Nm] -> Switch7/3
  VTQD_CreepBaseTqD_Nm/1 -> [VTQD_CreepBaseTqD_Nm]
  VTQD_CreepBaseTqR_Nm/1 -> [VTQD_CreepBaseTqR_Nm]
  VTQD_GearActualPosn_enum/1 -> [VTQD_GearActualPosn_enum]
  [VTQD_BOSReduction_gain] -> Relational Operator5/1
  NOT/1 -> AND/3
  [VVMC_APSActive_flg] -> NOT/1
  VVMC_APSActive_flg/1 -> [VVMC_APSActive_flg]
  VTQD_LowIdleAccPedal_flg/1 -> [VTQD_LowIdleAccPedal_flg]
  [VTQD_LowIdleAccPedal_flg] -> NOT2/1
  NOT2/1 -> AND/4
  [VTQD_BrkSwSta_flg] -> NOT3/1
  AND2/1 -> OR/3
  AND1/1 -> OR1/1
  Detect Change/1 -> OR1/2
  Relational Operator2/1 -> OR/1
  [VTQD_LowIdleAccPedal_flg] -> AND2/1
  [VTQD_GearActualPosn_enum] -> Detect Change/1
  NOT3/1 -> AND2/2
  SR_Latch/1 -> VTQD_BOSEnable_flg/1  "VTQD_BOSEnable_flg"
  AND/1 -> NOT1/1, SR_Latch/1
  [VTQD_HighBPSPosn_flg] -> OR/2
  OR/1 -> AND1/2
  NOT1/1 -> AND1/1
  [VTQD_PedalMapWhlTq_Nm] -> Relational Operator2/1
  [VTQD_BOSTq_Nm] -> Relational Operator2/2
  VTQD_BrkSwSta_flg/1 -> [VTQD_BrkSwSta_flg]
  VTQD_HighBPSPosn_flg/1 -> [VTQD_HighBPSPosn_flg]
  VTQD_LimpHomeAct_flg/1 -> [VTQD_LimpHomeAct_flg]
  Logical Operator13/1 -> OR2/2
  Constant96/1 -> Logical Operator13/2
  [VTQD_LimpHomeAct_flg] -> Logical Operator13/1
  OR1/1 -> OR2/1
  OR2/1 -> SR_Latch/2
